simulink model "QET_KV"  (R2015b)
settings: Solver=ode4  SolverMode=SingleTasking  StartTime=0.0  StopTime=inf  FixedStep=Ts  RelTol=1e-3
values from neighbouring files (symbols this model uses):
  F_M_Direction = [1 1 1 -1 -1 -1]    [Config_StepperMotor.m]
  NanoCal7342 = [-0.945276141167 14.673559188843 0.251662999392 -14.892200469971 -0.854624807835 0.034513175488 ... (first row only)    [NanoCalibration.m]
  Resolution = (360/200 * 1/64)    (= 0.028125)    [Config_StepperMotor.m]
undefined symbols (not defined in the file or in its folder): AnalogPos_to_deg, anVE, anVE_GBC_Kbi, anVE_GBC_Kbp, anVE_K_int, anVE_Position_Gain_inv, anVE_Saturation, B, Chirp_Amplitude, Chirp_Freq_Max, Chirp_Freq_Min, Chirp_Period, Chirp_Time_Start, Chirp_Type, delay, Delta, DO_DG409_A0, DO_DG409_A1, Driver_Type, HIL, K, K_gyro, Kd, Kp, lambda, mag, Pos_Final, Pos_Init, Pos_Threshold, PSoC_Freq, qc_get_step_size, Stabilization_Period, Test_type, Times, Torque_Threshold, Ts, Ts_loop, VE_Platform, VE_Type
libraries: quarc_library x22, simulink x13, dspsigops x1
(part 1 of 3)
settings Model: SimulationMode=external  ExtModeTrigDuration=1000000  Creator=17vall  LastModifiedBy=15lpds
settings SolverCC: PositivePriorityOrder=on  InsertRTBMode=Never (minimum delay)
settings DataIOCC: LimitDataPoints=off  SaveFormat=Array  SignalLoggingSaveFormat=ModelDataLogs
settings OptimizationCC: SimCompilerOptimization=on
settings DebuggingCC: SolverPrmCheckMsg=warning
settings HardwareCC: ProdBitPerPointer=32  ProdLargestAtomicFloat=None  ProdIntDivRoundTo=Undefined  ProdEndianess=Unspecified  ProdWordSize=32  ProdHWDeviceType=32-bit Generic
settings RTWCC: SystemTargetFile=quarc_win64.tlc  TemplateMakefile=quarc_default_tmf  Description=QUARC Win64 Target
settings STFCustomTargetCC: CombineOutputUpdateFcns=on  CPPClassGenCompliant=off  GRTInterface=off
settings GRTTargetCC: ParMdlRefBuildCompliant=off  CompOptLevelCompliant=off  GeneratePreprocessorConditionals=Disable all  MatFileLogging=off  CPPClassGenCompliant=off  UseToolchainInfoCompliant=off  ExtMode=on  ExtModeMexFile=quarc_comm
settings ConfigComp: CovModelRefEnable=Off  CovSFcnEnable=off

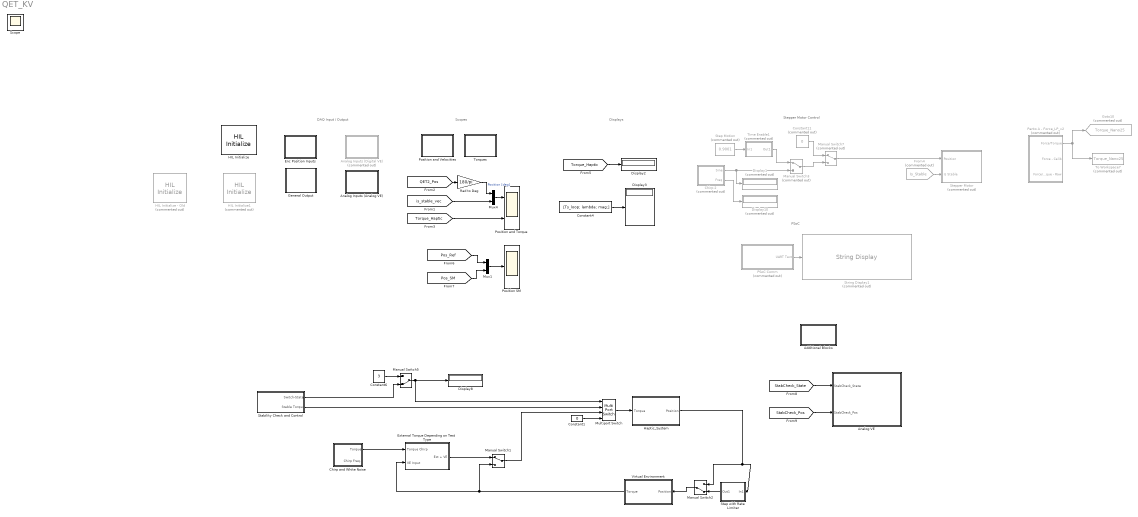
== system QET_KV ==
  note: Stepper Motor Control
  note: PSoC
  note: DAQ Input / Output
  note: Scopes
  note: Displays
  Additional Blocks : Subsystem
  Analog Inputs (Analog VE) : Subsystem
  Analog Inputs (Digital VE) : Subsystem  Commented=on
  Analog VE : Subsystem
  Chirp 2 : Subsystem  Commented=on
  Chirp and White Noise : Subsystem
  Constant1 : Constant  Value=0
  Constant11 : Constant  Commented=on  Value=0
  Constant4 : Constant  Value=[Ts_loop; lambda; mag;]
  Constant6 : Constant  Value=3
  Display1 : Display  Commented=on
  Display10 : Display  Commented=on
  Display2 : Display
  Display3 : Display
  Display8 : Display
  Enc Position Inputs : Subsystem
  External Torque Depending on Test Type : Subsystem
  From4 : From  Commented=on  GotoTag=Is_Stable  TagVisibility=global
  General Output : Subsystem
  Goto10 : Goto  Commented=on  GotoTag=Torque_Nano25  TagVisibility=global
  HIL Initialize : quarc_library/Data Acquisition/Generic/Configuration/HIL Initialize  Priority=-99  object_name=HIL-1  board_type=q8  board_number=0  board_options=""  exclusive=off  active=off  hardware_clocks=[0:1]  clock_modes=[0 0]  initial_clock_frequencies=[]  set_clock_params_at_start=on  set_clock_params_at_switch_in=off  set_clock_frequencies_at_start=off  set_clock_frequencies_at_switch_in=off  analog_input_channels=[0:7]  analog_input_maximums=10  analog_input_minimums=-10  set_analog_input_params_at_start=off  set_analog_input_params_at_switch_in=off  analog_output_channels=[0:7]  analog_output_maximums=[10]  analog_output_minimums=[-10]  initial_analog_outputs=[0]  final_analog_outputs=[0]  watchdog_analog_outputs=0  set_analog_output_params_at_start=on  set_analog_output_params_at_switch_in=off  set_analog_outputs_at_start=on  set_analog_outputs_at_switch_in=off  set_analog_outputs_at_terminate=on  set_analog_outputs_at_switch_out=off  set_analog_outputs_on_watchdog=off  digital_input_channels=[]  digital_output_channels=[0 7:15]  digital_output_configuration=[]  initial_digital_outputs=[0 1 0]  final_digital_outputs=[0 1 0]  watchdog_digital_outputs=[2]  set_digital_output_params_at_start=off  set_digital_output_params_at_switch_in=off  set_digital_outputs_at_start=on  set_digital_outputs_at_switch_in=off  set_digital_outputs_at_terminate=on  set_digital_outputs_at_switch_out=off  set_digital_outputs_on_watchdog=off  encoder_channels=[0:3]  quadrature=[0 0 4 4]  encoder_filter_frequency=(1/120e-9)/1  initial_encoder_counts=[0]  set_encoder_params_at_start=on  set_encoder_params_at_switch_in=off  set_encoder_counts_at_start=on  set_encoder_counts_at_switch_in=off  pwm_channels=[1]  pwm_modes=[1]  pwm_frequency=0.5  pwm_configuration=[]  pwm_alignment=[]  pwm_polarity=[]  pwm_leading_deadband=[]  pwm_trailing_deadband=[]  initial_pwm_outputs=[0]  final_pwm_outputs=[0]  watchdog_pwm_outputs=[]  set_pwm_params_at_start=on  set_pwm_params_at_switch_in=off  set_pwm_outputs_at_start=on  set_pwm_outputs_at_switch_in=off  set_pwm_outputs_at_terminate=on  set_pwm_outputs_at_switch_out=off  set_pwm_outputs_on_watchdog=off  other_output_channels=[]  initial_other_outputs=[]  final_other_outputs=[]  watchdog_other_outputs=[]  set_other_outputs_at_start=off  set_other_outputs_at_switch_in=off  set_other_outputs_at_terminate=off  set_other_outputs_at_switch_out=off  set_other_outputs_on_watchdog=off
  HIL Initialize - Old : quarc_library/Data Acquisition/Generic/Configuration/HIL Initialize  Priority=-99  Commented=on  object_name=HIL-1  board_type=q8  board_number=0  board_options=update_rate=normal;decimation=1  exclusive=off  active=off  hardware_clocks=[1]  clock_modes=[1]  initial_clock_frequencies=[]  set_clock_params_at_start=on  set_clock_params_at_switch_in=off  set_clock_frequencies_at_start=off  set_clock_frequencies_at_switch_in=off  analog_input_channels=[0:7]  analog_input_maximums=10  analog_input_minimums=-10  set_analog_input_params_at_start=off  set_analog_input_params_at_switch_in=off  analog_output_channels=[0:7]  analog_output_maximums=[10]  analog_output_minimums=[-10]  initial_analog_outputs=[0]  final_analog_outputs=[0]  watchdog_analog_outputs=0  set_analog_output_params_at_start=on  set_analog_output_params_at_switch_in=off  set_analog_outputs_at_start=on  set_analog_outputs_at_switch_in=off  set_analog_outputs_at_terminate=on  set_analog_outputs_at_switch_out=off  set_analog_outputs_on_watchdog=off  digital_input_channels=[]  digital_output_channels=[0 7 8:15]  digital_output_configuration=[]  initial_digital_outputs=[0 1 0]  final_digital_outputs=[0 1 0]  watchdog_digital_outputs=[2]  set_digital_output_params_at_start=off  set_digital_output_params_at_switch_in=off  set_digital_outputs_at_start=on  set_digital_outputs_at_switch_in=off  set_digital_outputs_at_terminate=on  set_digital_outputs_at_switch_out=off  set_digital_outputs_on_watchdog=off  encoder_channels=[0:3]  quadrature=[0 0 4 4]  encoder_filter_frequency=(1/120e-9)/1  initial_encoder_counts=[0]  set_encoder_params_at_start=on  set_encoder_params_at_switch_in=off  set_encoder_counts_at_start=on  set_encoder_counts_at_switch_in=off  pwm_channels=[1]  pwm_modes=[1]  pwm_frequency=0.5  pwm_configuration=[]  pwm_alignment=[]  pwm_polarity=[]  pwm_leading_deadband=[]  pwm_trailing_deadband=[]  initial_pwm_outputs=[0]  final_pwm_outputs=[0]  watchdog_pwm_outputs=[]  set_pwm_params_at_start=on  set_pwm_params_at_switch_in=off  set_pwm_outputs_at_start=on  set_pwm_outputs_at_switch_in=off  set_pwm_outputs_at_terminate=on  set_pwm_outputs_at_switch_out=off  set_pwm_outputs_on_watchdog=off  other_output_channels=[]  initial_other_outputs=[]  final_other_outputs=[]  watchdog_other_outputs=[]  set_other_outputs_at_start=off  set_other_outputs_at_switch_in=off  set_other_outputs_at_terminate=off  set_other_outputs_at_switch_out=off  set_other_outputs_on_watchdog=off
  HIL Initialize1 : quarc_library/Data Acquisition/Generic/Configuration/HIL Initialize  Priority=-99  Commented=on  object_name=HIL-3  board_type=q4  board_number=0  board_options=update_rate=normal;decimation=1  exclusive=off  active=off  hardware_clocks=[1]  clock_modes=[1]  initial_clock_frequencies=[]  set_clock_params_at_start=on  set_clock_params_at_switch_in=off  set_clock_frequencies_at_start=off  set_clock_frequencies_at_switch_in=off  analog_input_channels=[0:3]  analog_input_maximums=10  analog_input_minimums=-10  set_analog_input_params_at_start=off  set_analog_input_params_at_switch_in=off  analog_output_channels=[0:3]  analog_output_maximums=[10]  analog_output_minimums=[-10]  initial_analog_outputs=[0]  final_analog_outputs=[0]  watchdog_analog_outputs=0  set_analog_output_params_at_start=on  set_analog_output_params_at_switch_in=off  set_analog_outputs_at_start=on  set_analog_outputs_at_switch_in=off  set_analog_outputs_at_terminate=on  set_analog_outputs_at_switch_out=off  set_analog_outputs_on_watchdog=off  digital_input_channels=[]  digital_output_channels=[0 7:8 13:15 9:10 12 11 6]  digital_output_configuration=[]  initial_digital_outputs=[0]  final_digital_outputs=[0]  watchdog_digital_outputs=[2]  set_digital_output_params_at_start=off  set_digital_output_params_at_switch_in=off  set_digital_outputs_at_start=on  set_digital_outputs_at_switch_in=off  set_digital_outputs_at_terminate=on  set_digital_outputs_at_switch_out=off  set_digital_outputs_on_watchdog=off  encoder_channels=[0:3]  quadrature=[0 0 4 4]  encoder_filter_frequency=(1/60e-9)/1  initial_encoder_counts=[0 0 0 0]  set_encoder_params_at_start=on  set_encoder_params_at_switch_in=off  set_encoder_counts_at_start=on  set_encoder_counts_at_switch_in=off  pwm_channels=[1]  pwm_modes=[1]  pwm_frequency=0.5  pwm_configuration=[]  pwm_alignment=[]  pwm_polarity=[]  pwm_leading_deadband=[]  pwm_trailing_deadband=[]  initial_pwm_outputs=[0]  final_pwm_outputs=[0]  watchdog_pwm_outputs=[]  set_pwm_params_at_start=on  set_pwm_params_at_switch_in=off  set_pwm_outputs_at_start=on  set_pwm_outputs_at_switch_in=off  set_pwm_outputs_at_terminate=on  set_pwm_outputs_at_switch_out=off  set_pwm_outputs_on_watchdog=off  other_output_channels=[]  initial_other_outputs=[]  final_other_outputs=[]  watchdog_other_outputs=[]  set_other_outputs_at_start=off  set_other_outputs_at_switch_in=off  set_other_outputs_at_terminate=off  set_other_outputs_at_switch_out=off  set_other_outputs_on_watchdog=off
  Haptic_System : Subsystem
  Manual Switch1 : ManualSwitch
  Manual Switch2 : ManualSwitch  CurrentSetting=0
  Manual Switch3 : ManualSwitch  Commented=on
  Manual Switch5 : ManualSwitch  CurrentSetting=0
  Manual Switch7 : ManualSwitch  Commented=on
  Multiport Switch : MultiPortSwitch  Inputs=2  DataPortForDefault=Additional data port  SampleTime=Ts
  Mux1 : Mux  Inputs=2
  Mux4 : Mux  Inputs=2
  PSoC Comm : Subsystem  Commented=on
  Panto A - Force_LP_v2 : Subsystem  Commented=on
  Position SM : Scope
  Position and Torque : Scope  NumInputPorts=2
  Position and Velocities : Subsystem
  Rad to Deg : Gain  Gain=180/pi
  Stability Check and Control : Subsystem
  Step Motion : Constant  Commented=on  Value=0.9001
  Step with Rate Limiter : Subsystem
  Stepper Motor : Subsystem  Commented=on
  String Display1 : quarc_library/Strings/String Display  Commented=on  alignment=left  display_mode=Console  sample_time=-1
  Time Enable1 : Subsystem  Commented=on
  To Workspace7 : ToWorkspace  Commented=on  VariableName=Torque_Nano25  SampleTime=-1
      settings: Save2DSignal=2-D array (concatenate along first dimension)
  Torques : Subsystem
  Virtual Environment : Subsystem
  Scope : Scope
  wires:
  Multiport Switch/1 -> Haptic_System/1(Torque)
  Constant1/1 -> Multiport Switch/4
  Constant4/1 -> Display3/1
  Rad to Deg/1 -> Mux4/1  "Position [deg]"
  Constant6/1 -> Manual Switch5/1
  Manual Switch5/1 -> Display8/1, Multiport Switch/1
  PSoC Comm/1(UART Text) -> String Display1/1
  Chirp 2/2(Freq) -> Display10/1
  Manual Switch7/1 -> Stepper Motor/1(Position)
  Chirp 2/1(Sine) -> Display1/1, Manual Switch3/2
  Constant11/1 -> Manual Switch7/1
  [is_stable_vec] -> Mux4/2
  [QET2_Pos] -> Rad to Deg/1
  [Torque_Haptic] -> Position and Torque/2
  Mux4/1 -> Position and Torque/1
  Haptic_System/1(Position) -> Step with Rate Limiter/1(In1), Manual Switch2/1
  Manual Switch1/1 -> Multiport Switch/3
  Virtual Environment/1(Torque) -> External Torque Depending on Test Type/2(VE Input), Manual Switch1/2
  Stability Check and Control/2(Stable Torque) -> Multiport Switch/2
  Stability Check and Control/1(Switch-State) -> Manual Switch5/2
  [Torque_Haptic] -> Display2/1
  Panto A - Force_LP_v2/1(Force/Torque) -> To Workspace7/1, Goto10/1
  From4/1 -> Stepper Motor/2(Is Stable)
  Mux1/1 -> Position SM/1
  [Pos_SM] -> Mux1/2
  [Pos_Ref] -> Mux1/1
  [StabCheck_State] -> Analog VE/1("StabCheck_State ")
  [StabCheck_Pos] -> Analog VE/2(StabCheck_Pos)
  Manual Switch2/1 -> Virtual Environment/1(Position)
  Step with Rate Limiter/1(Out1) -> Manual Switch2/2
  Chirp and White Noise/1(Torque) -> External Torque Depending on Test Type/1(Torque Chirp)
  External Torque Depending on Test Type/1(Ext + VE) -> Manual Switch1/1
  Step Motion/1 -> Time Enable1/1(In1)
  Manual Switch3/1 -> Manual Switch7/2
  Time Enable1/1(Out1) -> Manual Switch3/1

== system QET_KV/Additional Blocks ==
  Computation Time : quarc_library/Sources/Time/Computation Time  Commented=on  sample_time=qc_get_step_size  use_model=on
  Display7 : Display  Commented=on
  Mux5 : Mux  Commented=on  Inputs=2
  Sample Time : quarc_library/Sources/Time/Sample Time  Priority=-99  Commented=on  sample_time=qc_get_step_size
  To Workspace6 : ToWorkspace  Commented=on  VariableName=Tc_vec  SampleTime=-1
      settings: Save2DSignal=2-D array (concatenate along first dimension)
  wires:
  Computation Time/1 -> Mux5/1
  Sample Time/1 -> Mux5/2
  Mux5/1 -> Display7/1, To Workspace6/1

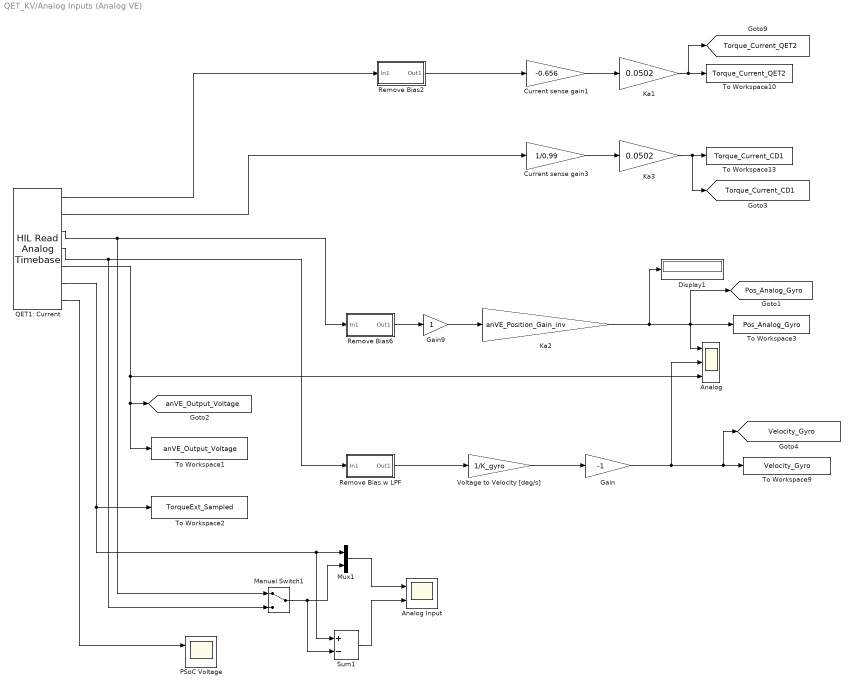
== system QET_KV/Analog Inputs (Analog VE) ==
  Analog : Scope  NumInputPorts=3
  "Analog Input " : Scope  NumInputPorts=2
  Current sense gain1 : Gain  Gain=-0.656  SampleTime=qc_get_step_size
  Current sense gain3 : Gain  Gain=1/0.99  SampleTime=qc_get_step_size
  Display1 : Display
  Gain : Gain  Gain=-1  SampleTime=qc_get_step_size
  Gain9 : Gain
  Ka1 : Gain  Gain=0.0502  SampleTime=qc_get_step_size
  Ka2 : Gain  Gain=anVE_Position_Gain_inv  SampleTime=qc_get_step_size
  Ka3 : Gain  Gain=0.0502  SampleTime=qc_get_step_size
  Manual Switch1 : ManualSwitch
  Mux1 : Mux  Inputs=2
  "PSoC Voltage " : Scope  NumInputPorts=2
  QET1: Current : quarc_library/Data Acquisition/Generic/Timebases/HIL Read Analog Timebase  object_name=HIL-1  clock=[0]  channels=[3 2 1 0 4 7 5]  samples_in_buffer=max(ceil(1/qc_get_step_size), 1)  active=on  vector_output=off
      settings: AttributesFormatString=(%<object_name>)
  Remove Bias w LPF : Subsystem
  Remove Bias2 : Subsystem
  Remove Bias6 : Subsystem
  Sum1 : Sum  Inputs=+-
  To Workspace1 : ToWorkspace  VariableName=anVE_Output_Voltage  SampleTime=-1
      settings: Save2DSignal=2-D array (concatenate along first dimension)
  To Workspace10 : ToWorkspace  VariableName=Torque_Current_QET2  SampleTime=-1
      settings: Save2DSignal=2-D array (concatenate along first dimension)
  To Workspace13 : ToWorkspace  VariableName=Torque_Current_CD1  SampleTime=-1
      settings: Save2DSignal=2-D array (concatenate along first dimension)
  To Workspace2 : ToWorkspace  VariableName=TorqueExt_Sampled  SampleTime=-1
      settings: Save2DSignal=2-D array (concatenate along first dimension)
  To Workspace3 : ToWorkspace  VariableName=Pos_Analog_Gyro  SampleTime=-1
      settings: Save2DSignal=2-D array (concatenate along first dimension)
  To Workspace9 : ToWorkspace  VariableName=Velocity_Gyro  SampleTime=-1
      settings: Save2DSignal=2-D array (concatenate along first dimension)
  Voltage to Velocity [deg/s] : Gain  Gain=1/K_gyro  SampleTime=qc_get_step_size
  tag scope: Pos_Analog_Gyro=global, Torque_Current_CD1=global, Torque_Current_QET2=global, Velocity_Gyro=global, anVE_Output_Voltage=global
  wires:
  QET1: Current/1 -> Remove Bias2/1(In1)
  Ka1/1 -> [Torque_Current_QET2], To Workspace10/1
  Current sense gain1/1 -> Ka1/1
  Remove Bias2/1(Out1) -> Current sense gain1/1
  Current sense gain3/1 -> Ka3/1
  Ka3/1 -> [Torque_Current_CD1], To Workspace13/1
  Remove Bias w LPF/1(Out1) -> Voltage to Velocity [deg/s]/1
  Gain/1 -> Analog/2, [Velocity_Gyro], To Workspace9/1
  Voltage to Velocity [deg/s]/1 -> Gain/1
  QET1: Current/3 -> Manual Switch1/1, Remove Bias6/1(In1)
  Ka2/1 -> Display1/1, Analog/1, To Workspace3/1, [Pos_Analog_Gyro]
  Remove Bias6/1(Out1) -> Gain9/1
  Gain9/1 -> Ka2/1
  QET1: Current/2 -> Current sense gain3/1
  QET1: Current/5 -> [anVE_Output_Voltage], To Workspace1/1, Analog/3
  Sum1/1 -> "Analog Input "/2
  Mux1/1 -> "Analog Input "/1
  QET1: Current/6 -> To Workspace2/1, Sum1/1, Mux1/1
  Manual Switch1/1 -> Sum1/2, Mux1/2
  QET1: Current/4 -> Manual Switch1/2, Remove Bias w LPF/1(In1)
  QET1: Current/7 -> "PSoC Voltage "/1

== system QET_KV/Analog Inputs (Digital VE) ==
  Current sense gain1 : Gain  Gain=-0.656  SampleTime=qc_get_step_size
  Current sense gain2 : Gain  Gain=2.2  SampleTime=qc_get_step_size
  Current sense gain3 : Gain  Gain=1/0.99  SampleTime=qc_get_step_size
  Deg to Rad2 : Gain  Gain=pi/180
  Gain : Gain  Gain=-1  SampleTime=qc_get_step_size
  Ka1 : Gain  Gain=0.0502  SampleTime=qc_get_step_size
  Ka2 : Gain  Gain=0.0502  SampleTime=qc_get_step_size
  Ka3 : Gain  Gain=0.0502  SampleTime=qc_get_step_size
  QET1: Current : quarc_library/Data Acquisition/Generic/Timebases/HIL Read Analog Timebase  object_name=HIL-1  clock=[0]  channels=[3 2 1 0]  samples_in_buffer=max(ceil(1/qc_get_step_size), 1)  active=on  vector_output=off
      settings: AttributesFormatString=(%<object_name>)
  Remove Bias w LPF : Subsystem
  Remove Bias2 : Subsystem
  Remove Bias5 : Subsystem
  Remove Bias6 : Subsystem
  To Workspace10 : ToWorkspace  VariableName=Torque_Current_QET2  SampleTime=-1
      settings: Save2DSignal=2-D array (concatenate along first dimension)
  To Workspace13 : ToWorkspace  VariableName=Torque_Current_CD1  SampleTime=-1
      settings: Save2DSignal=2-D array (concatenate along first dimension)
  To Workspace5 : ToWorkspace  VariableName=Torque_Current_AMC  SampleTime=-1
      settings: Save2DSignal=2-D array (concatenate along first dimension)
  To Workspace9 : ToWorkspace  VariableName=Velocity_Gyro  SampleTime=-1
      settings: Save2DSignal=2-D array (concatenate along first dimension)
  Voltage to Velocity : Gain  Gain=1/K_gyro  SampleTime=qc_get_step_size
  tag scope: Torque_Current_AMC=global, Torque_Current_CD1=global, Torque_Current_QET2=global, Velocity_Gyro=global
  wires:
  QET1: Current/1 -> Remove Bias2/1(In1)
  Ka1/1 -> [Torque_Current_QET2], To Workspace10/1
  Current sense gain1/1 -> Ka1/1
  Remove Bias2/1(Out1) -> Current sense gain1/1
  Current sense gain2/1 -> Ka2/1
  Ka2/1 -> [Torque_Current_AMC], To Workspace5/1
  Remove Bias5/1(Out1) -> Current sense gain2/1
  Current sense gain3/1 -> Ka3/1
  Ka3/1 -> [Torque_Current_CD1], To Workspace13/1
  Remove Bias6/1(Out1) -> Current sense gain3/1
  QET1: Current/4 -> Remove Bias w LPF/1(In1)
  Voltage to Velocity/1 -> Deg to Rad2/1
  Remove Bias w LPF/1(Out1) -> Voltage to Velocity/1
  Gain/1 -> [Velocity_Gyro], To Workspace9/1
  Deg to Rad2/1 -> Gain/1
  QET1: Current/2 -> Remove Bias6/1(In1)
  QET1: Current/3 -> Remove Bias5/1(In1)

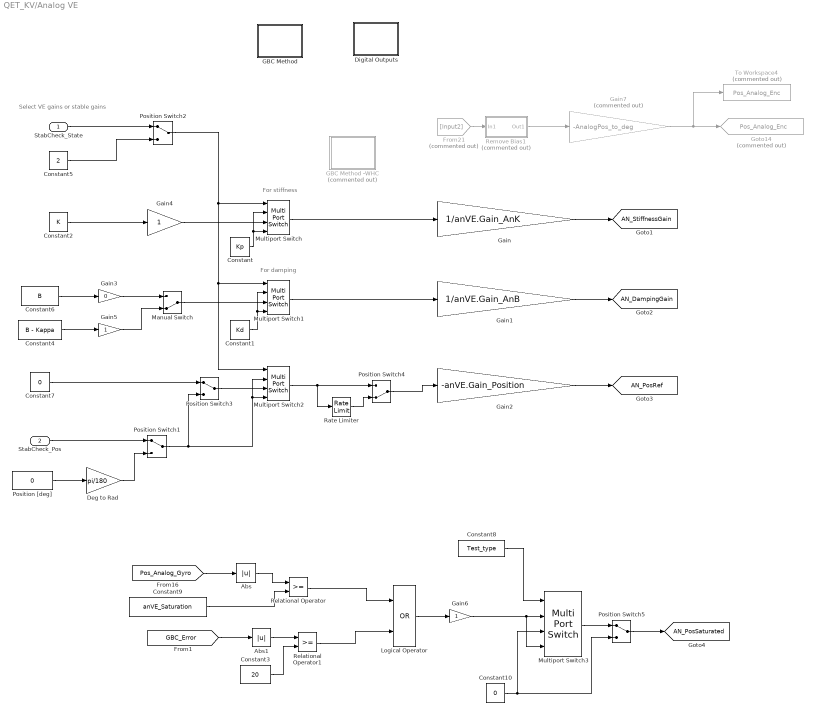
== system QET_KV/Analog VE ==
  note: For stiffness
  note: For damping
  note: Select VE gains or stable gains
  "StabCheck_State " : Inport
  StabCheck_Pos : Inport  Port=2
  Abs : Abs
  Abs1 : Abs
  Constant : Constant  Value=Kp
  Constant1 : Constant  Value=Kd
  Constant10 : Constant  Value=0
  Constant2 : Constant  Value=K
  Constant3 : Constant  Value=20
  Constant4 : Constant  Value=B - Kappa
  Constant5 : Constant  Value=2
  Constant6 : Constant  Value=B
  Constant7 : Constant  Value=0
  Constant8 : Constant  Value=Test_type
  Constant9 : Constant  Value=anVE_Saturation
  Deg to Rad : Gain  Gain=pi/180
  Digital Outputs : Subsystem
  From21 : From  Commented=on  GotoTag=Input2  TagVisibility=global
  GBC Method : Subsystem
  GBC Method -WHC : Subsystem  Commented=on
  Gain : Gain  Gain=1/anVE.Gain_AnK
  Gain1 : Gain  Gain=1/anVE.Gain_AnB
  Gain2 : Gain  Gain=-anVE.Gain_Position
  Gain3 : Gain  Gain=0
  Gain4 : Gain
  Gain5 : Gain
  Gain6 : Gain
  Gain7 : Gain  Commented=on  Gain=-AnalogPos_to_deg
  Goto14 : Goto  Commented=on  GotoTag=Pos_Analog_Enc  TagVisibility=global
  Logical Operator : Logic  Operator=OR  AllPortsSameDT=off  OutDataTypeStr=boolean
  Manual Switch : ManualSwitch  CurrentSetting=0
  Multiport Switch : MultiPortSwitch  Inputs=2  DataPortForDefault=Additional data port  SampleTime=Ts
  Multiport Switch1 : MultiPortSwitch  Inputs=2  DataPortForDefault=Additional data port  SampleTime=Ts
  Multiport Switch2 : MultiPortSwitch  Inputs=2  DataPortForDefault=Additional data port  SampleTime=Ts
  Multiport Switch3 : MultiPortSwitch  DataPortOrder=Specify indices  Inputs=2  DataPortIndices={[1,2,3,5],4}  DataPortForDefault=Additional data port  SampleTime=Ts
  Position Switch{1..3,5} (4 alike) : ManualSwitch
  Position Switch4 : ManualSwitch  CurrentSetting=0
  Position [deg] : Constant  Value=0
  Rate Limiter : RateLimiter  RisingSlewLimit=100 * pi/180  FallingSlewLimit=-100 * pi/180  SampleTimeMode=inherited
  Relational Operator : RelationalOperator  OutDataTypeStr=boolean
  Relational Operator1 : RelationalOperator  OutDataTypeStr=boolean
  Remove Bias1 : Subsystem  Commented=on
  To Workspace4 : ToWorkspace  Commented=on  VariableName=Pos_Analog_Enc  SampleTime=-1
      settings: Save2DSignal=2-D array (concatenate along first dimension)
  tag scope: AN_DampingGain=global, AN_PosRef=global, AN_PosSaturated=global, AN_StiffnessGain=global
  wires:
  From21/1 -> Remove Bias1/1(In1)
  Gain7/1 -> To Workspace4/1, Goto14/1
  Remove Bias1/1(Out1) -> Gain7/1
  Constant/1 -> Multiport Switch/2, Multiport Switch/4
  Constant1/1 -> Multiport Switch1/2, Multiport Switch1/4
  Multiport Switch/1 -> Gain/1
  Multiport Switch1/1 -> Gain1/1
  Gain/1 -> [AN_StiffnessGain]
  Gain1/1 -> [AN_DampingGain]
  Gain2/1 -> [AN_PosRef]
  Constant4/1 -> Gain5/1
  Manual Switch/1 -> Multiport Switch1/3
  Position [deg]/1 -> Deg to Rad/1
  Deg to Rad/1 -> Position Switch1/2
  "StabCheck_State "/1 -> Position Switch2/1
  Position Switch2/1 -> Multiport Switch/1, Multiport Switch2/1, Multiport Switch1/1
  Constant5/1 -> Position Switch2/2
  Gain3/1 -> Manual Switch/1
  Constant6/1 -> Gain3/1
  Gain4/1 -> Multiport Switch/3
  Constant2/1 -> Gain4/1
  Gain5/1 -> Manual Switch/2
  [Pos_Analog_Gyro] -> Abs/1
  Constant9/1 -> Relational Operator/2
  Abs/1 -> Relational Operator/1
  Logical Operator/1 -> Gain6/1
  Relational Operator/1 -> Logical Operator/1
  Relational Operator1/1 -> Logical Operator/2
  Abs1/1 -> Relational Operator1/1
  Constant3/1 -> Relational Operator1/2
  [GBC_Error] -> Abs1/1
  Position Switch1/1 -> Multiport Switch2/2, Multiport Switch2/4, Position Switch3/2
  Position Switch3/1 -> Multiport Switch2/3
  Constant7/1 -> Position Switch3/1
  Constant8/1 -> Multiport Switch3/1
  Gain6/1 -> Multiport Switch3/4, Multiport Switch3/2
  Constant10/1 -> Multiport Switch3/3, Position Switch5/2
  Rate Limiter/1 -> Position Switch4/2
  Multiport Switch2/1 -> Rate Limiter/1, Position Switch4/1
  Position Switch4/1 -> Gain2/1
  StabCheck_Pos/1 -> Position Switch1/1
  Multiport Switch3/1 -> Position Switch5/1
  Position Switch5/1 -> [AN_PosSaturated]

== system QET_KV/Chirp 2 ==
  Clock : Clock
  Constant1 : Constant  Value=Chirp_Freq_Min
  Constant2 : Constant  Value=Chirp_Freq_Max
  Constant3 : Constant  Value=Chirp_Period
  Constant4 : Constant  Value=Chirp_Time_Start
  Constant5 : Constant  Value=Chirp_Type
  Constant6 : Constant  Value=Chirp_Amplitude
  MATLAB Function : MATLAB Function  TreatAsAtomicUnit=on
  Manual Switch : ManualSwitch  CurrentSetting=0
  Product1 : Product
  Step : Step  Time=Times(3)  Before=1  After=0
  Transfer Fcn1 : TransferFcn  Denominator=[1/(2*pi*1) 1]
  Sine : Outport
  Freq : Outport  Port=2
  wires:
  Constant2/1 -> MATLAB Function/7(fmax)
  Clock/1 -> MATLAB Function/2(clock)
  Constant1/1 -> MATLAB Function/6(fmin)
  Constant3/1 -> MATLAB Function/3(chirp_period)
  MATLAB Function/2(f) -> Freq/1
  Constant4/1 -> MATLAB Function/4(chirp_start)
  Constant5/1 -> MATLAB Function/1(type)
  Constant6/1 -> MATLAB Function/5(chirp_amp)
  Step/1 -> Transfer Fcn1/1
  Transfer Fcn1/1 -> Product1/2
  Manual Switch/1 -> Sine/1
  Product1/1 -> Manual Switch/2
  MATLAB Function/1(y) -> Manual Switch/1, Product1/1

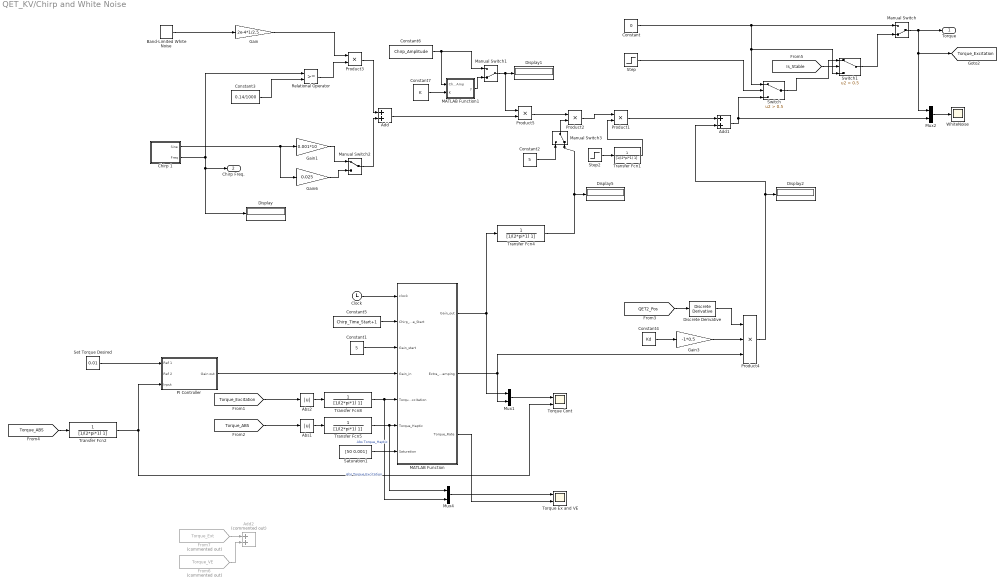
== system QET_KV/Chirp and White Noise ==
  Abs1 : Abs
  Abs2 : Abs
  Add : Sum
  Add1 : Sum
  Add2 : Sum  Commented=on
  Band-Limited White Noise : simulink/Sources/Band-Limited White Noise  Cov=[0.1]  Ts=qc_get_step_size  seed=[23341]
  Chirp 1 : Subsystem
  Clock : Clock
  Constant : Constant  Value=0
  Constant1 : Constant  Value=5
  Constant2 : Constant  Value=5
  Constant3 : Constant  Value=0.14/1000
  Constant4 : Constant  Value=Kd
  Constant5 : Constant  Value=Chirp_Time_Start+1
  Constant6 : Constant  Value=Chirp_Amplitude
  Constant7 : Constant  Value=K
  Discrete Derivative : simulink/Discrete/Discrete Derivative  gainval=1.0  ICPrevScaledInput=0.0  InputProcessing=Inherited  OutMin=[]  OutMax=[]  OutDataType=fixdt(1, 16)  OutScaling=2^-10  DoSatur=off
  Display{,1..2,5} (4 alike) : Display
  From6 : From  Commented=on  GotoTag=Torque_VE  TagVisibility=global
  From7 : From  Commented=on  GotoTag=Torque_Ext  TagVisibility=global
  Gain : Gain  Gain=2e-4*1/2.5
  Gain1 : Gain  Gain=0.001*10  SampleTime=qc_get_step_size
  Gain3 : Gain  Gain=-1*0.5
  Gain6 : Gain  Gain=0.025  SampleTime=qc_get_step_size
  MATLAB Function : MATLAB Function  TreatAsAtomicUnit=on
  MATLAB Function1 : MATLAB Function  TreatAsAtomicUnit=on
  Manual Switch : ManualSwitch  CurrentSetting=0
  Manual Switch1 : ManualSwitch  CurrentSetting=0
  Manual Switch2 : ManualSwitch
  Manual Switch3 : ManualSwitch  CurrentSetting=0
  Mux1 : Mux  Inputs=2
  Mux2 : Mux  Inputs=2
  Mux4 : Mux  Inputs=2
  PI Controller : Subsystem
  Product{1..3,5} (4 alike) : Product
  Product4 : Product  Inputs=3
  Relational Operator : RelationalOperator  OutDataTypeStr=boolean
  Saturation1 : Constant  Value=[50 0.001]
  Set Torque Desired : Constant  Value=0.01
  Step : Step  Time=Chirp_Time_Start  Before=1  After=0
  Step2 : Step  Time=Times(3)  Before=1  After=0
  Switch : Switch  Criteria=u2 > Threshold  Threshold=0.5
  Switch1 : Switch  Criteria=u2 > Threshold  Threshold=0.5
  Torque Cont : Scope  NumInputPorts=2
  Torque Ex and VE : Scope  NumInputPorts=2
  Transfer Fcn{1..2,4..5,8} (5 alike) : TransferFcn  Denominator=[1/(2*pi*1) 1]
  WhiteNoise : Scope
  Torque : Outport
  Chirp Freq. : Outport  Port=2
  tag scope: Torque_Excitation=global
  wires:
  Constant/1 -> Manual Switch/1, Switch1/3, Switch/1
  Band-Limited White Noise/1 -> Gain/1
  Step/1 -> Switch/2
  Chirp 1/1(Sine) -> Gain1/1, Gain6/1
  Manual Switch/1 -> [Torque_Excitation], Mux2/1, Torque/1
  Step2/1 -> Transfer Fcn1/1
  Transfer Fcn1/1 -> Product1/2
  Add/1 -> Product5/2
  Mux2/1 -> WhiteNoise/1
  Manual Switch2/1 -> Add/2
  [Torque_ABS] -> Transfer Fcn2/1
  Product2/1 -> Product1/1
  Product5/1 -> Product2/1
  Transfer Fcn2/1 -> Torque Cont/2, PI Controller/3(Input)
  Switch/1 -> Switch1/1
  Switch1/1 -> Manual Switch/2
  [Is_Stable] -> Switch1/2
  Gain1/1 -> Manual Switch2/1
  Gain6/1 -> Manual Switch2/2
  Manual Switch3/1 -> Product2/2
  Constant2/1 -> Manual Switch3/1
  Chirp 1/2(Freq) -> Chirp Freq./1, Display/1, Relational Operator/1
  Gain/1 -> Product3/1
  Product3/1 -> Add/1
  Relational Operator/1 -> Product3/2
  Constant3/1 -> Relational Operator/2
  Transfer Fcn4/1 -> Display5/1, Manual Switch3/2
  Saturation1/1 -> MATLAB Function/7(Saturation)
  Constant5/1 -> MATLAB Function/2(Chirp_Time_Start)
  Clock/1 -> MATLAB Function/1(clock)
  Constant1/1 -> MATLAB Function/3(Gain_start)
  Abs1/1 -> Transfer Fcn5/1
  Transfer Fcn5/1 -> Mux4/1, MATLAB Function/6(Torque_Haptic)  "Abs Torque_Haptic"
  Mux4/1 -> Torque Ex and VE/1
  Set Torque Desired/1 -> PI Controller/1(Ref 1)
  PI Controller/1(Gain out) -> MATLAB Function/4(Gain_in)
  Abs2/1 -> Transfer Fcn8/1
  [Torque_Excitation] -> Abs2/1
  Transfer Fcn8/1 -> Mux4/2, MATLAB Function/5(Torque_Excitation)  "Abs Torque Excitation"
  MATLAB Function/3(Torque_Rate) -> Torque Ex and VE/2
  Discrete Derivative/1 -> Product4/1
  MATLAB Function/2(Extra_Damping) -> Product4/3, Mux1/2
  Add1/1 -> Mux2/2, Switch/3
  Product1/1 -> Add1/1
  Product4/1 -> Display2/1, Add1/2
  [QET2_Pos] -> Discrete Derivative/1
  Constant4/1 -> Gain3/1
  Gain3/1 -> Product4/2
  MATLAB Function/1(Gain_out) -> Transfer Fcn4/1, Mux1/1
  Mux1/1 -> Torque Cont/1
  Manual Switch1/1 -> Display1/1, Product5/1
  Constant6/1 -> MATLAB Function1/1(Chirp_Amp), Manual Switch1/1
  MATLAB Function1/1(y) -> Manual Switch1/2
  Constant7/1 -> MATLAB Function1/2(K)
  [Torque_ABS] -> Abs1/1
  From6/1 -> Add2/2
  From7/1 -> Add2/1

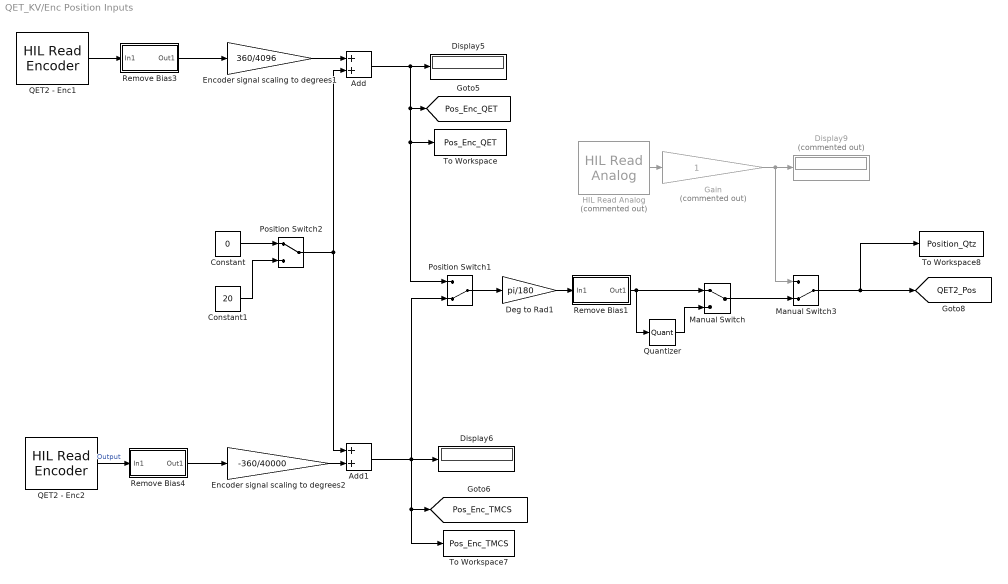
== system QET_KV/Enc Position Inputs ==
  Add : Sum
  Add1 : Sum
  Constant : Constant  Value=0
  Constant1 : Constant  Value=20
  Deg to Rad1 : Gain  Gain=pi/180
  Display5 : Display
  Display6 : Display
  Display9 : Display  Commented=on
  Encoder signal scaling to degrees1 : Gain  Gain=360/4096
  Encoder signal scaling to degrees2 : Gain  Gain=-360/40000
  "Gain " : Gain  Commented=on
  HIL Read Analog : quarc_library/Data Acquisition/Generic/Immediate I//O/HIL Read Analog  Commented=on  object_name=HIL-1  channels=0  sample_time=qc_get_step_size  active=on  vector_output=off
  Manual Switch : ManualSwitch
  Manual Switch3 : ManualSwitch  CurrentSetting=0
  Position Switch1 : ManualSwitch  CurrentSetting=0
  Position Switch2 : ManualSwitch
  QET2 - Enc1 : quarc_library/Data Acquisition/Generic/Immediate I//O/HIL Read Encoder  object_name=HIL-1  channels=[3]  sample_time=qc_get_step_size  active=on  vector_output=off  data_type_mode=Inherit via back propagation  data_type=double
  QET2 - Enc2 : quarc_library/Data Acquisition/Generic/Immediate I//O/HIL Read Encoder  object_name=HIL-1  channels=[2]  sample_time=qc_get_step_size  active=on  vector_output=off  data_type_mode=Inherit via back propagation  data_type=double
  Quantizer : Quantizer  QuantizationInterval=(360/(1024*4)) * pi/180  LinearizeAsGain=off
  Remove Bias1 : Subsystem
  Remove Bias3 : Subsystem
  Remove Bias4 : Subsystem
  To Workspace : ToWorkspace  VariableName=Pos_Enc_QET  SampleTime=-1
      settings: Save2DSignal=2-D array (concatenate along first dimension)
  To Workspace7 : ToWorkspace  VariableName=Pos_Enc_TMCS  SampleTime=-1
      settings: Save2DSignal=2-D array (concatenate along first dimension)
  To Workspace8 : ToWorkspace  VariableName=Position_Qtz  SaveFormat=Structure With Time  SampleTime=-1
      settings: Save2DSignal=2-D array (concatenate along first dimension)
  tag scope: Pos_Enc_QET=global, Pos_Enc_TMCS=global, QET2_Pos=global
  wires:
  Position Switch1/1 -> Deg to Rad1/1
  Add1/1 -> To Workspace7/1, [Pos_Enc_TMCS], Display6/1, Position Switch1/2
  Add/1 -> Display5/1, Position Switch1/1, To Workspace/1, [Pos_Enc_QET]
  Deg to Rad1/1 -> Remove Bias1/1(In1)
  Remove Bias1/1(Out1) -> Quantizer/1, Manual Switch/1
  QET2 - Enc1/1 -> Remove Bias3/1(In1)
  QET2 - Enc2/1 -> Remove Bias4/1(In1)  "Output"
  Remove Bias3/1(Out1) -> Encoder signal scaling to degrees1/1
  Remove Bias4/1(Out1) -> Encoder signal scaling to degrees2/1
  Quantizer/1 -> Manual Switch/2
  HIL Read Analog/1 -> "Gain "/1
  Manual Switch3/1 -> To Workspace8/1, [QET2_Pos]
  Manual Switch/1 -> Manual Switch3/2
  "Gain "/1 -> Display9/1, Manual Switch3/1
  Encoder signal scaling to degrees1/1 -> Add/1
  Encoder signal scaling to degrees2/1 -> Add1/2
  Constant/1 -> Position Switch2/1
  Constant1/1 -> Position Switch2/2
  Position Switch2/1 -> Add1/1, Add/2

== system QET_KV/External Torque Depending on Test Type ==
  Torque Chirp : Inport
  VE Input : Inport  Port=2
  Add : Sum
  Constant : Constant  Value=0
  Constant2 : Constant  Value=Test_type
  Multiport Switch1 : MultiPortSwitch  DataPortOrder=Specify indices  Inputs=2  DataPortIndices={1,[2,5]}  DataPortForDefault=Additional data port  SampleTime=Ts
  Multiport Switch2 : MultiPortSwitch  DataPortOrder=Specify indices  Inputs=2  DataPortIndices={5,1}  SampleTime=Ts
  To Workspace4 : ToWorkspace  VariableName=Torque_Ext  SampleTime=-1
      settings: Save2DSignal=2-D array (concatenate along first dimension)
  Ext + VE : Outport
  tag scope: Torque_Ext=global
  wires:
  Torque Chirp/1 -> Multiport Switch1/3
  Multiport Switch1/1 -> To Workspace4/1, [Torque_Ext], Add/1, Multiport Switch2/2
  Constant/1 -> Multiport Switch1/2, Multiport Switch1/4
  Constant2/1 -> Multiport Switch2/1, Multiport Switch1/1
  VE Input/1 -> Add/2
  Multiport Switch2/1 -> Ext + VE/1
  Add/1 -> Multiport Switch2/3

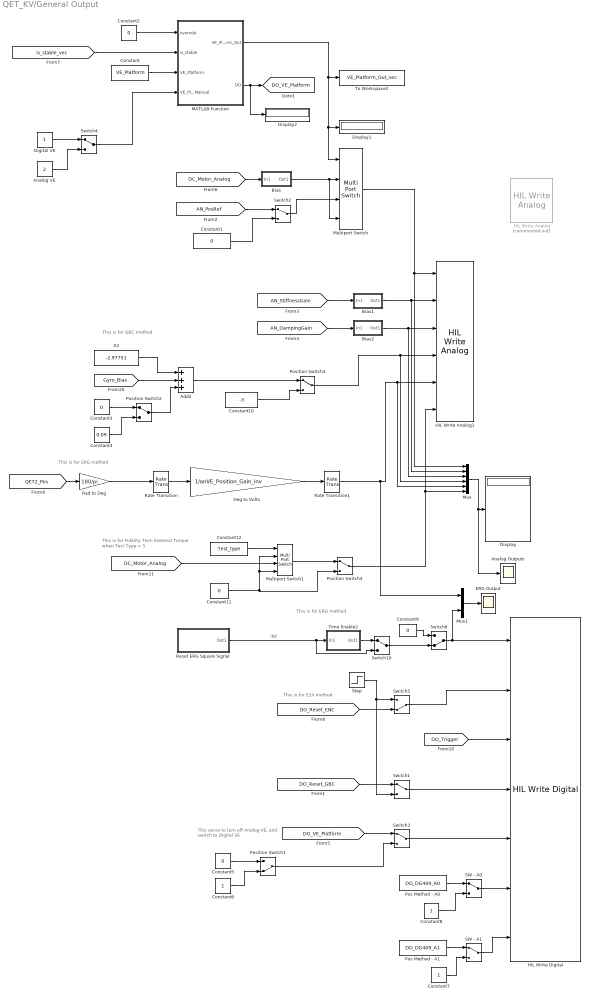
== system QET_KV/General Output ==
  note: This is for GBC method
  note: This is for ERG method
  note: This serve to turn off Analog VE,
      |  and switch to Digital VE
  note: This is for ERG method
  note: This is for E2A method
  note: This is  for Fidelity Test:
      | External Torque when Test Type = 5
  Add2 : Sum  Inputs=+++
  Analog Outputs : Scope
  Analog VE : Constant  Value=2
  Bias : Subsystem
  Bias1 : Subsystem
  Bias2 : Subsystem
  Constant : Constant  Value=VE_Platform
  Constant{1..3,5,9,11} (6 alike) : Constant  Value=0
  Constant10 : Constant  Value=-3
  Constant12 : Constant  Value=Test_type
  Constant4 : Constant  Value=0.09
  Constant6 : Constant
  Constant7 : Constant
  Constant8 : Constant
  Deg to Volts : Gain  Gain=1/anVE_Position_Gain_inv
  Digital VE : Constant
  Display : Display
  Display1 : Display
  Display2 : Display
  ERG Output : Scope
  HIL Write Analog : quarc_library/Data Acquisition/Generic/Immediate I//O/HIL Write Analog  Commented=on  object_name=HIL-1  channels=[0 2]  sample_time=qc_get_step_size  active=off  vector_input=off
  HIL Write Analog1 : quarc_library/Data Acquisition/Generic/Immediate I//O/HIL Write Analog  object_name=HIL-1  channels=[0:5]  sample_time=qc_get_step_size  active=off  vector_input=off
  HIL Write Digital : quarc_library/Data Acquisition/Generic/Immediate I//O/HIL Write Digital  object_name=HIL-1  channels=[10:11 13:15 8:9]  sample_time=-1  active=off  vector_input=off
  MATLAB Function : MATLAB Function  TreatAsAtomicUnit=on
  Multiport Switch : MultiPortSwitch  DataPortOrder=Specify indices  Inputs=2  DataPortIndices={1,2}  DataPortForDefault=Additional data port  SampleTime=Ts
  Multiport Switch1 : MultiPortSwitch  DataPortOrder=Specify indices  Inputs=2  DataPortIndices={1,5}  DataPortForDefault=Additional data port  SampleTime=Ts
  Mux : Mux  Inputs=6
  Mux1 : Mux  Inputs=2
  Pos Method - A0 : Constant  Value=DO_DG409_A0
  Pos Method - A1 : Constant  Value=DO_DG409_A1
  Position Switch1 : ManualSwitch  CurrentSetting=0
  Position Switch2 : ManualSwitch
  Position Switch3 : ManualSwitch
  Position Switch4 : ManualSwitch
  Rad to Deg : Gain  Gain=180/pi
  Rate Transition : RateTransition  Integrity=off  Deterministic=off  OutPortSampleTime=Ts_loop
  Rate Transition1 : RateTransition  Integrity=off  Deterministic=off  OutPortSampleTime=Ts
  Reset ERG Square Signal : Subsystem
  SW - A0 : ManualSwitch
  SW - A1 : ManualSwitch
  Step : Step  Time=2  SampleTime=Ts
  Switch{1..4,10} (5 alike) : ManualSwitch
  Switch5 : ManualSwitch  CurrentSetting=0
  Switch6 : ManualSwitch  CurrentSetting=0
  Time Enable2 : Subsystem
  To Workspace2 : ToWorkspace  VariableName=VE_Platform_Out_vec  SampleTime=-1
      settings: Save2DSignal=2-D array (concatenate along first dimension)
  X2 : Constant  Value=-2.97751
  tag scope: DO_VE_Platform=global
  wires:
  [DC_Motor_Analog] -> Bias/1(In1)
  X2/1 -> Add2/1
  [Gyro_Bias] -> Add2/2
  Bias/1(Out1) -> Multiport Switch/2, Multiport Switch/4
  Multiport Switch/1 -> Mux/1, HIL Write Analog1/1
  [AN_StiffnessGain] -> Bias1/1(In1)
  [AN_DampingGain] -> Bias2/1(In1)
  Bias1/1(Out1) -> Mux/2, HIL Write Analog1/2
  Bias2/1(Out1) -> Mux/3, HIL Write Analog1/3
  Switch2/1 -> Multiport Switch/3
  [AN_PosRef] -> Switch2/1
  Constant1/1 -> Switch2/2
  Mux/1 -> Analog Outputs/1, Display/1
  [is_stable_vec] -> MATLAB Function/2(is_stable)
  Digital VE/1 -> Switch4/1
  Analog VE/1 -> Switch4/2
  Switch4/1 -> MATLAB Function/4(VE_Platform_Manual)
  Constant2/1 -> MATLAB Function/1(override)
  Constant/1 -> MATLAB Function/3(VE_Platform)
  MATLAB Function/1(VE_Platform_Out) -> To Workspace2/1, Multiport Switch/1, Display1/1
  MATLAB Function/2(DO) -> Display2/1, [DO_VE_Platform]
  Constant3/1 -> Position Switch2/1
  Constant4/1 -> Position Switch2/2
  Position Switch2/1 -> Add2/3
  [DO_VE_Platform] -> Switch3/1
  Constant5/1 -> Position Switch1/1
  Constant6/1 -> Position Switch1/2
  Position Switch1/1 -> Switch3/2
  [DO_Reset_ENC] -> Switch5/2
  [QET2_Pos] -> Rad to Deg/1
  Rad to Deg/1 -> Rate Transition/1
  Reset ERG Square Signal/1(Out1) -> Time Enable2/1(In1), Switch10/2  "IN2"
  Time Enable2/1(Out1) -> Switch10/1
  Switch10/1 -> Switch6/2
  Constant9/1 -> Switch6/1
  Switch6/1 -> Mux1/2, HIL Write Digital/1
  Add2/1 -> Position Switch3/1
  Position Switch3/1 -> Mux/4, HIL Write Analog1/4
  Constant10/1 -> Position Switch3/2
  Deg to Volts/1 -> Rate Transition1/1
  Step/1 -> Switch5/1, Switch1/2
  [DO_Reset_GBC] -> Switch1/1
  Switch3/1 -> HIL Write Digital/5
  Switch1/1 -> HIL Write Digital/4
  Switch5/1 -> HIL Write Digital/2
  [DO_Trigger] -> HIL Write Digital/3
  SW - A0/1 -> HIL Write Digital/6
  SW - A1/1 -> HIL Write Digital/7
  Pos Method - A0/1 -> SW - A0/1
  Constant8/1 -> SW - A0/2
  Pos Method - A1/1 -> SW - A1/1
  Constant7/1 -> SW - A1/2
  Position Switch4/1 -> Mux/6, HIL Write Analog1/6
  Constant11/1 -> Position Switch4/2, Multiport Switch1/4, Multiport Switch1/2
  Constant12/1 -> Multiport Switch1/1
  [DC_Motor_Analog] -> Multiport Switch1/3
  Multiport Switch1/1 -> Position Switch4/1
  Rate Transition1/1 -> Mux1/1, Mux/5, HIL Write Analog1/5
  Rate Transition/1 -> Deg to Volts/1
  Mux1/1 -> ERG Output/1

== system QET_KV/Haptic_System ==
  Torque : Inport
  Constant7 : Constant  Value=Driver_Type
  Discrete Derivative : simulink/Discrete/Discrete Derivative  gainval=1.0  ICPrevScaledInput=0.0  InputProcessing=Inherited  OutMin=[]  OutMax=[]  OutDataType=fixdt(1, 16)  OutScaling=2^-10  DoSatur=off
  Driver Voltage or Current : Subsystem
  Mux2 : Mux  Inputs=2
  Power : Scope  Commented=on
  Product : Product  Inputs=**  SampleTime=Ts
  Rate Transition : RateTransition  Integrity=off  OutPortSampleTime=Ts*2
  Rate Transition1 : RateTransition  Integrity=off  OutPortSampleTime=Ts
  To Workspace2 : ToWorkspace  VariableName=Power_k  SampleTime=-1
      settings: Save2DSignal=2-D array (concatenate along first dimension)
  Transfer Fcn1 : TransferFcn  Denominator=[1/(2*pi*150/3) 1]
  Voltage1 : Scope
  Position : Outport
  tag scope: DC_Motor_Analog=global, QET2_Power_k=global, Torque_Haptic=global
  wires:
  Torque/1 -> [Torque_Haptic], Driver Voltage or Current/1(Torque), Product/2
  [QET2_Pos] -> Rate Transition/1
  Discrete Derivative/1 -> Rate Transition1/1
  Rate Transition/1 -> Discrete Derivative/1
  Rate Transition1/1 -> Transfer Fcn1/1
  Product/1 -> To Workspace2/1, Power/1, [QET2_Power_k]
  Transfer Fcn1/1 -> Product/1
  [QET2_Pos] -> Position/1
  Mux2/1 -> Voltage1/1
  Driver Voltage or Current/1(Output) -> [DC_Motor_Analog], Mux2/1
  Driver Voltage or Current/2(Output (Not Saturated)) -> Mux2/2
  Constant7/1 -> Driver Voltage or Current/2(Type)

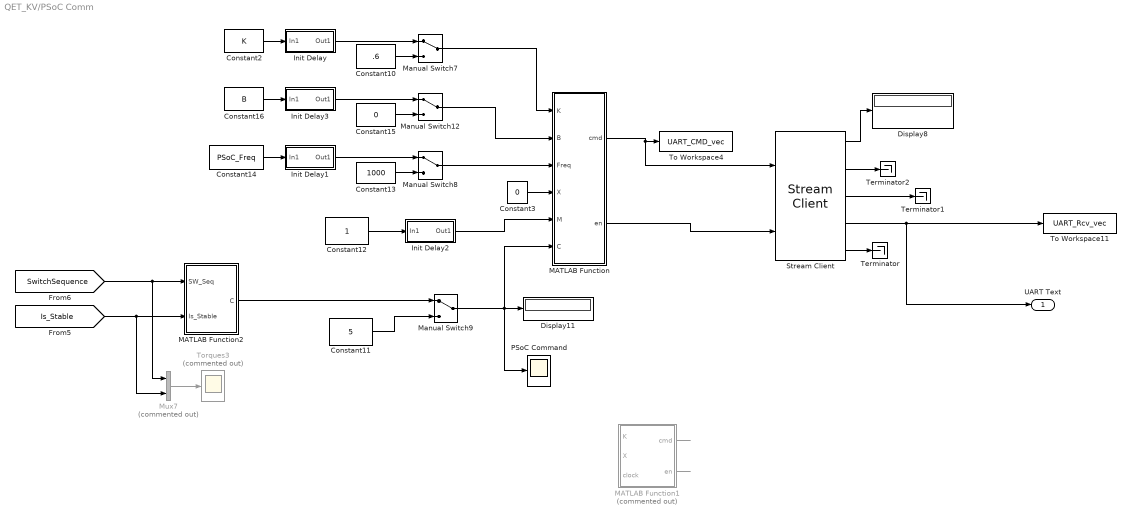
== system QET_KV/PSoC Comm ==
  Constant10 : Constant  Value=.6
  Constant11 : Constant  Value=5
  Constant12 : Constant
  Constant13 : Constant  Value=1000
  Constant14 : Constant  Value=PSoC_Freq
  Constant15 : Constant  Value=0
  Constant16 : Constant  Value=B
  Constant2 : Constant  Value=K
  Constant3 : Constant  Value=0
  Display11 : Display
  Display8 : Display
  Init Delay : Subsystem
  Init Delay1 : Subsystem
  Init Delay2 : Subsystem
  Init Delay3 : Subsystem
  MATLAB Function : MATLAB Function  TreatAsAtomicUnit=on
  MATLAB Function1 : MATLAB Function  Commented=on  TreatAsAtomicUnit=on
  MATLAB Function2 : MATLAB Function  TreatAsAtomicUnit=on  SystemSampleTime=qc_get_step_size
  Manual Switch{7..9,12} (4 alike) : ManualSwitch
  Mux7 : Mux  Commented=on  Inputs=2
  PSoC Command : Scope
  Stream Client : quarc_library/Communications/Basic/Stream Client  uri_source=Specify via dialog (do not evaluate)  uri=serial://localhost:10?baud='115200'  apply_uri_to_all_configs=on  send_buffer_size=1460  receive_buffer_size=1460  byte_order=little endian (Intel - LSB first)  optimization=Minimum latency  implementation=Use blocking I/O in a separate thread  send_options=Send all data  receive_options=Receive all data  send_fifo_size=1000  receive_fifo_size=1000  send_priority=0  receive_priority=0  default_value=[0]  send_dimensions=off  receive_dimensions=off  max_dimensions=-1  sample_time=qc_get_step_size  active=off  data_type=Inherited via back propagation  type_expr=BusObject
      settings: AttributesFormatString="\"serial://localhost:10?baud='115200'\""
  Terminator : Terminator
  Terminator1 : Terminator
  Terminator2 : Terminator
  To Workspace11 : ToWorkspace  VariableName=UART_Rcv_vec  SampleTime=-1
      settings: Save2DSignal=2-D array (concatenate along first dimension)
  To Workspace4 : ToWorkspace  VariableName=UART_CMD_vec  SampleTime=-1
      settings: Save2DSignal=2-D array (concatenate along first dimension)
  Torques3 : Scope  Commented=on
  UART Text : Outport
  wires:
  Stream Client/4 -> UART Text/1, To Workspace11/1
  Stream Client/1 -> Display8/1
  MATLAB Function/2(en) -> Stream Client/2
  MATLAB Function/1(cmd) -> Stream Client/1, To Workspace4/1
  Constant3/1 -> MATLAB Function/4(X)
  Stream Client/5 -> Terminator/1
  Stream Client/3 -> Terminator1/1
  Stream Client/2 -> Terminator2/1
  Manual Switch7/1 -> MATLAB Function/1(K)
  Constant10/1 -> Manual Switch7/2
  Constant12/1 -> Init Delay2/1(In1)
  Manual Switch9/1 -> PSoC Command/1, Display11/1, MATLAB Function/6(C)
  Constant2/1 -> Init Delay/1(In1)
  Init Delay/1(Out1) -> Manual Switch7/1
  Constant13/1 -> Manual Switch8/2
  Constant14/1 -> Init Delay1/1(In1)
  Init Delay1/1(Out1) -> Manual Switch8/1
  Init Delay2/1(Out1) -> MATLAB Function/5(M)
  Manual Switch8/1 -> MATLAB Function/3(Freq)
  Constant11/1 -> Manual Switch9/2
  [Is_Stable] -> Mux7/2, MATLAB Function2/2(Is_Stable)
  [SwitchSequence] -> Mux7/1, MATLAB Function2/1(SW_Seq)
  Mux7/1 -> Torques3/1
  MATLAB Function2/1(C) -> Manual Switch9/1
  Manual Switch12/1 -> MATLAB Function/2(B)
  Constant15/1 -> Manual Switch12/2
  Constant16/1 -> Init Delay3/1(In1)
  Init Delay3/1(Out1) -> Manual Switch12/1
  MATLAB Function1/1(cmd) -> ?
  MATLAB Function1/2(en) -> ?

== system QET_KV/Panto A - Force_LP_v2 ==
  note: Version 2
  note: Forces / Torques
  Axis Selector1 : Subsystem
  Axis Selector2 : Subsystem  Commented=on
  Discrete Filters : Subsystem
  DocBlock : simulink/Model-Wide Utilities/DocBlock  DocumentType=Text
      content=|
      | Type your documentation here
  Force1 : Scope  Commented=on
  Gain : Gain  Gain=NanoCal7342  Multiplication=Matrix(K*u)
  HIL Initialize : quarc_library/Data Acquisition/Generic/Configuration/HIL Initialize  object_name=HIL-2  board_type=ni_pci_6034e  board_number=0  board_options=update_rate=normal;decimation=1  exclusive=off  active=off  hardware_clocks=[]  clock_modes=[]  initial_clock_frequencies=[]  set_clock_params_at_start=off  set_clock_params_at_switch_in=off  set_clock_frequencies_at_start=off  set_clock_frequencies_at_switch_in=off  analog_input_channels=[0:5]  analog_input_maximums=10  analog_input_minimums=-10  set_analog_input_params_at_start=on  set_analog_input_params_at_switch_in=off  analog_output_channels=[]  analog_output_maximums=[]  analog_output_minimums=[]  initial_analog_outputs=[]  final_analog_outputs=[]  watchdog_analog_outputs=[]  set_analog_output_params_at_start=off  set_analog_output_params_at_switch_in=off  set_analog_outputs_at_start=off  set_analog_outputs_at_switch_in=off  set_analog_outputs_at_terminate=off  set_analog_outputs_at_switch_out=off  set_analog_outputs_on_watchdog=off  digital_input_channels=[]  digital_output_channels=[]  digital_output_configuration=[]  initial_digital_outputs=[1]  final_digital_outputs=[1]  watchdog_digital_outputs=[]  set_digital_output_params_at_start=off  set_digital_output_params_at_switch_in=off  set_digital_outputs_at_start=on  set_digital_outputs_at_switch_in=off  set_digital_outputs_at_terminate=on  set_digital_outputs_at_switch_out=off  set_digital_outputs_on_watchdog=off  encoder_channels=[]  quadrature=[0]  encoder_filter_frequency=[]  initial_encoder_counts=[0]  set_encoder_params_at_start=off  set_encoder_params_at_switch_in=off  set_encoder_counts_at_start=on  set_encoder_counts_at_switch_in=off  pwm_channels=[]  pwm_modes=[0]  pwm_frequency=20e6/4096  pwm_configuration=[]  pwm_alignment=[]  pwm_polarity=[]  pwm_leading_deadband=[]  pwm_trailing_deadband=[]  initial_pwm_outputs=[0]  final_pwm_outputs=[0]  watchdog_pwm_outputs=[]  set_pwm_params_at_start=on  set_pwm_params_at_switch_in=off  set_pwm_outputs_at_start=on  set_pwm_outputs_at_switch_in=off  set_pwm_outputs_at_terminate=on  set_pwm_outputs_at_switch_out=off  set_pwm_outputs_on_watchdog=off  other_output_channels=[]  initial_other_outputs=[]  final_other_outputs=[]  watchdog_other_outputs=[]  set_other_outputs_at_start=off  set_other_outputs_at_switch_in=off  set_other_outputs_at_terminate=off  set_other_outputs_at_switch_out=off  set_other_outputs_on_watchdog=off
  HIL Read Analog : quarc_library/Data Acquisition/Generic/Immediate I//O/HIL Read Analog  object_name=HIL-2  channels=[0:5]  sample_time=qc_get_step_size  active=on  vector_output=on
  HIL Read Analog1 : quarc_library/Data Acquisition/Generic/Immediate I//O/HIL Read Analog  Commented=on  object_name=HIL-2  channels=[0:5]  sample_time=qc_get_step_size  active=on  vector_output=on
  Product : Product  RndMeth=Zero
  Sample and Hold : dspsigops/Sample and Hold  trig=Rising edge  initCond=0  latchinput=off
  Step : Step  Time=0.3  SampleTime=0
  Sum : Sum  Inputs=|+-
  Force/Torque : Outport
  Force - Calib : Outport  Port=2
  Force/Torque - Raw : Outport  Port=3
  wires:
  HIL Read Analog/1 -> Gain/1, Force/Torque - Raw/1
  Step/1 -> Sample and Hold/Trigger, Product/2
  Sample and Hold/1 -> Sum/2
  Gain/1 -> Discrete Filters/1(Input [6x1]), Force - Calib/1
  Sum/1 -> Axis Selector1/1(Forces [6x1])
  Axis Selector1/1(Forces [3x1]) -> Product/1
  Product/1 -> Force/Torque/1
  Discrete Filters/1(Output [6x1]) -> Sum/1, Sample and Hold/1
  HIL Read Analog1/1 -> Force1/1

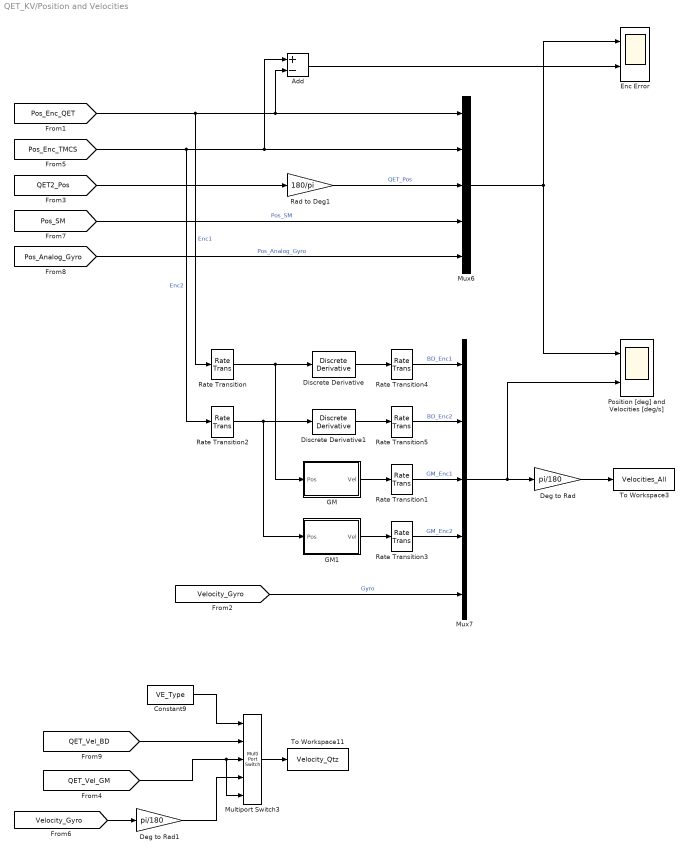
== system QET_KV/Position and Velocities ==
  Add : Sum  Inputs=+-
  Constant9 : Constant  Value=VE_Type
  Deg to Rad : Gain  Gain=pi/180
  Deg to Rad1 : Gain  Gain=pi/180
  Discrete Derivative : simulink/Discrete/Discrete Derivative  gainval=1.0  ICPrevScaledInput=0.0  InputProcessing=Inherited  OutMin=[]  OutMax=[]  OutDataType=fixdt(1, 16)  OutScaling=2^-10  DoSatur=off
  Discrete Derivative1 : simulink/Discrete/Discrete Derivative  gainval=1.0  ICPrevScaledInput=0.0  InputProcessing=Inherited  OutMin=[]  OutMax=[]  OutDataType=fixdt(1, 16)  OutScaling=2^-10  DoSatur=off
  Enc Error : Scope  NumInputPorts=2
  GM : Subsystem
  GM1 : Subsystem
  Multiport Switch3 : MultiPortSwitch  DataPortForDefault=Additional data port  SampleTime=Ts
  Mux6 : Mux  Inputs=5
  Mux7 : Mux  Inputs=5
  Position [deg] and Velocities [deg/s] : Scope  NumInputPorts=2
  Rad to Deg1 : Gain  Gain=180/pi
  Rate Transition : RateTransition  Integrity=off  Deterministic=off  OutPortSampleTime=Ts_loop
  Rate Transition{1,3..5} (4 alike) : RateTransition  Integrity=off  Deterministic=off  OutPortSampleTime=Ts
  Rate Transition2 : RateTransition  Integrity=off  Deterministic=off  OutPortSampleTime=Ts_loop
  To Workspace11 : ToWorkspace  VariableName=Velocity_Qtz  SampleTime=-1
      settings: Save2DSignal=2-D array (concatenate along first dimension)
  To Workspace3 : ToWorkspace  VariableName=Velocities_All  SampleTime=-1
      settings: Save2DSignal=2-D array (concatenate along first dimension)
  wires:
  [Pos_Enc_QET] -> Rate Transition/1, Add/2, Mux6/1  "Enc1"
  GM1/1(Vel) -> Rate Transition3/1
  GM/1(Vel) -> Rate Transition1/1
  Rate Transition2/1 -> GM1/1(Pos), Discrete Derivative1/1
  Rate Transition/1 -> GM/1(Pos), Discrete Derivative/1
  [Pos_Enc_TMCS] -> Rate Transition2/1, Add/1, Mux6/2  "Enc2"
  Discrete Derivative/1 -> Rate Transition4/1
  Discrete Derivative1/1 -> Rate Transition5/1
  Rate Transition4/1 -> Mux7/1  "BD_Enc1"
  Rate Transition5/1 -> Mux7/2  "BD_Enc2"
  Rate Transition3/1 -> Mux7/4  "GM_Enc2"
  Rate Transition1/1 -> Mux7/3  "GM_Enc1"
  Mux6/1 -> Enc Error/1, Position [deg] and Velocities [deg/s]/1
  Mux7/1 -> Position [deg] and Velocities [deg/s]/2, Deg to Rad/1
  Deg to Rad/1 -> To Workspace3/1
  [Velocity_Gyro] -> Mux7/5  "Gyro"
  [QET2_Pos] -> Rad to Deg1/1
  Rad to Deg1/1 -> Mux6/3  "QET_Pos"
  Multiport Switch3/1 -> To Workspace11/1
  [QET_Vel_BD] -> Multiport Switch3/2
  [QET_Vel_GM] -> Multiport Switch3/5, Multiport Switch3/3
  [Velocity_Gyro] -> Deg to Rad1/1
  Constant9/1 -> Multiport Switch3/1
  Add/1 -> Enc Error/2
  [Pos_SM] -> Mux6/4  "Pos_SM"
  [Pos_Analog_Gyro] -> Mux6/5  "Pos_Analog_Gyro"
  Deg to Rad1/1 -> Multiport Switch3/4
